simulink model "pendulo_optimo"  (R2017b)
settings: Solver=ode3  StartTime=0.0  StopTime=inf  FixedStep=h  RelTol=1e-3  EnableMultiTasking=on
values from neighbouring files (symbols this model uses):
  h = 0.001    [LQR_Ganancias.m]    (also in LQR_Ganancias2.m)
undefined symbols (not defined in the file or in its folder): National_Instruments, PCI
libraries: sldrtlib x4, fuzblock x1
settings Model: SimulationMode=external  Creator=Jovani  LastModifiedBy=js231
settings DataIOCC: LimitDataPoints=on  SaveFormat=Array
settings OptimizationCC: LifeSpan=inf
settings DebuggingCC: UnderspecifiedInitializationDetection=Classic  MergeDetectMultiDrivingBlocksExec=none  SolverPrmCheckMsg=warning  StateNameClashWarn=warning  SFUnexpectedBacktrackingDiag=warning  SFNoUnconditionalDefaultTransitionDiag=warning  SFExecutionAtInitializationDiag=none
settings HardwareCC: TargetBitPerLong=64  TargetBitPerPointer=64  TargetIntDivRoundTo=Zero  TargetEndianess=LittleEndian  TargetWordSize=64  TargetHWDeviceType=Intel->x86-64
settings ModelReferenceCC: PropagateSignalLabelsOutOfModel=off
settings RTWCC: SystemTargetFile=sldrt.tlc  TemplateMakefile=sldrt.tmf  Description=Simulink Desktop Real-Time  RTWCompilerOptimization=on
settings CodeAppCC: MaxIdLength=95  StateflowObjectComments=on
settings SimulinkDesktopRealTimeCC: TargetPreCompLibLocation=C:\Program Files\MATLAB\R2017b\toolbox\sldrt\lib\win64  TargetLangStandard=C89/C90 (ANSI)  SupportVariableSizeSignals=off
settings ConfigComp: CovMetricSettings=dw  CovHtmlReporting=on  CovSaveCumulativeToWorkspaceVar=on  CovSaveSingleToWorkspaceVar=on  CovExternalEMLEnable=off

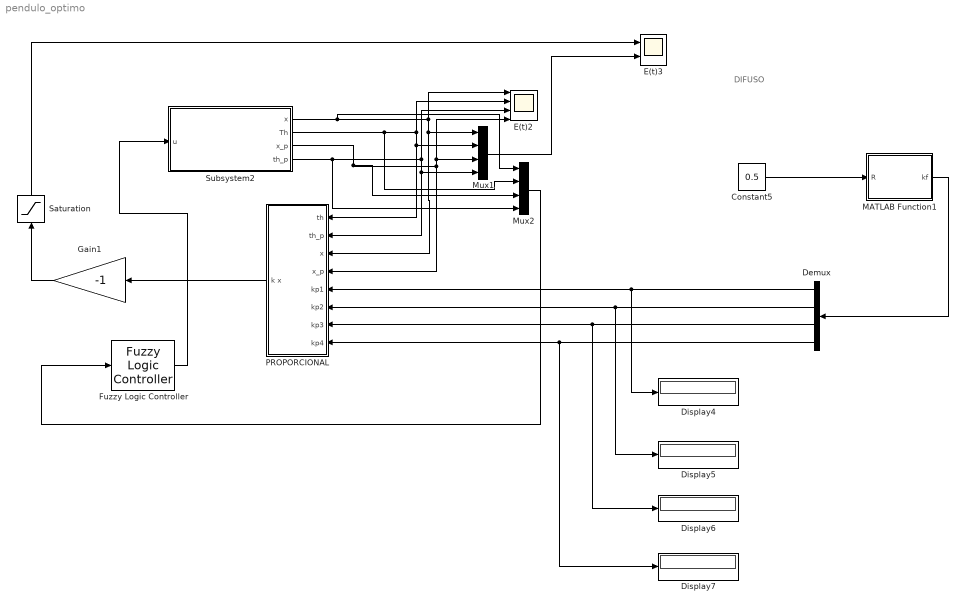
== system pendulo_optimo ==
  note: DIFUSO
  Constant5 : Constant  Value=0.5
  Demux : Demux
  Display{4..7} (4 alike) : Display
  E(t)2 : Scope  NumInputPorts=4
  E(t)3 : Scope  NumInputPorts=2
  Fuzzy Logic Controller : fuzblock/Fuzzy Logic  Controller  FIS=TS_carro_pendulo  OutputSampleNumber=101  DataType=double  FuzzifiedInputs=off  RuleFiringStrengths=off  RuleOutputs=off  AggregatedOutputs=off  SimulateUsing=Interpreted execution
  Gain1 : Gain  Gain=-1
  MATLAB Function1 : MATLAB Function  TreatAsAtomicUnit=on
  Mux1 : Mux
  Mux2 : Mux
  PROPORCIONAL : Subsystem
  Saturation : Saturate  UpperLimit=7.5  LowerLimit=-7.5
  Subsystem2 : Subsystem
  wires:
  Gain1/1 -> Saturation/1
  Subsystem2/4(th_p) -> Mux2/4, PROPORCIONAL/2(th_p), Mux1/4, E(t)2/3
  Subsystem2/3(x_p) -> Mux2/3, E(t)2/4, Mux1/3, PROPORCIONAL/4(x_p)
  Subsystem2/2(Th) -> Mux2/2, Mux1/2, PROPORCIONAL/1(th), E(t)2/2
  Subsystem2/1(x) -> Mux2/1, Mux1/1, PROPORCIONAL/3(x), E(t)2/1
  Mux1/1 -> E(t)3/2
  PROPORCIONAL/1(k x) -> Gain1/1
  Saturation/1 -> E(t)3/1
  Constant5/1 -> MATLAB Function1/1(R)
  MATLAB Function1/1(kf) -> Demux/1
  Demux/1 -> Display4/1, PROPORCIONAL/5(kp1)
  Demux/2 -> Display5/1, PROPORCIONAL/6(kp2)
  Demux/3 -> Display6/1, PROPORCIONAL/7(kp3)
  Demux/4 -> Display7/1, PROPORCIONAL/8(kp4)
  Mux2/1 -> Fuzzy Logic Controller/1
  Fuzzy Logic Controller/1 -> Subsystem2/1(u)

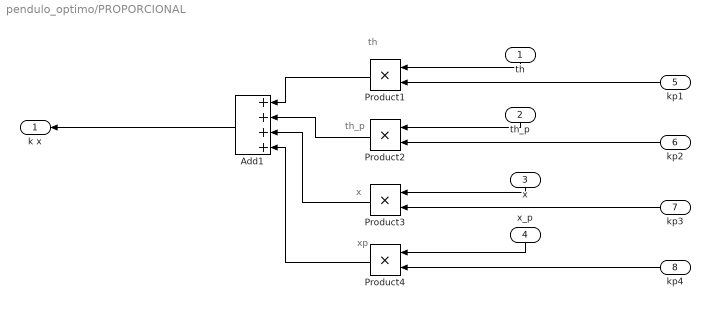
== system pendulo_optimo/PROPORCIONAL ==
  note: xp
  note: x
  note: th_p
  note: th
  th : Inport
  th_p : Inport  Port=2
  x : Inport  Port=3
  x_p : Inport  Port=4
  kp1 : Inport  Port=5
  kp2 : Inport  Port=6
  kp3 : Inport  Port=7
  kp4 : Inport  Port=8
  Add1 : Sum  Inputs=++++
  Product{1..4} (4 alike) : Product
  k x : Outport
  wires:
  x_p/1 -> Product4/1
  x/1 -> Product3/1
  th_p/1 -> Product2/1
  th/1 -> Product1/1
  Add1/1 -> k x/1
  Product4/1 -> Add1/4
  Product3/1 -> Add1/3
  Product2/1 -> Add1/2
  Product1/1 -> Add1/1
  kp3/1 -> Product3/2
  kp1/1 -> Product1/2
  kp2/1 -> Product2/2
  kp4/1 -> Product4/2

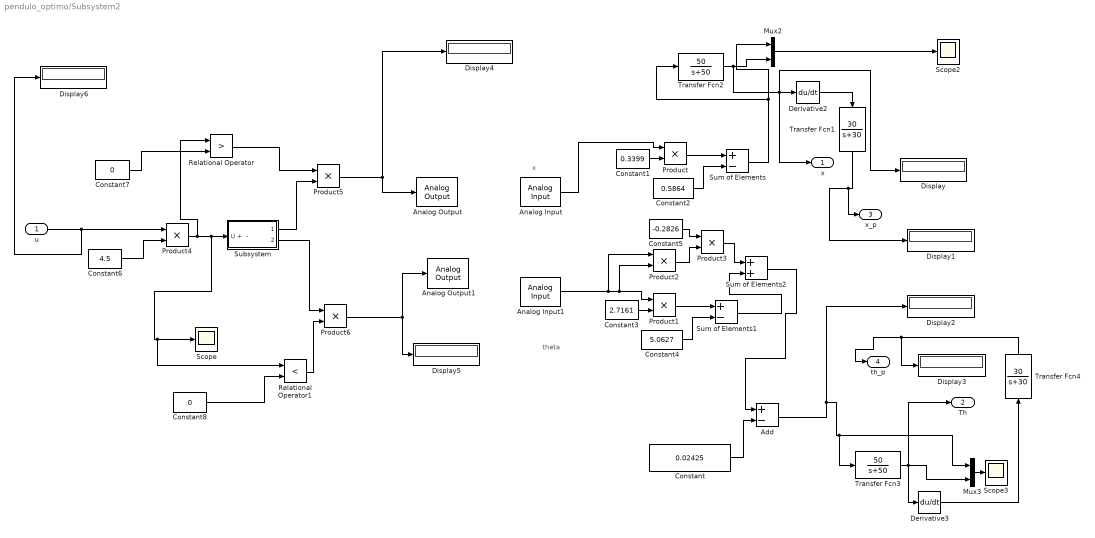
== system pendulo_optimo/Subsystem2 ==
  note: x
  note: theta
  u : Inport
  Add : Sum  Inputs=+-
  Analog Input : sldrtlib/Analog Input  SampleTime=h  MaxMissedTicks=10  ShowMissedTicks=off  YieldWhenWaiting=off  DrvName=National_Instruments/PCI-6071E  DrvAddress=0  DrvOptions=[0 0 0 0 0 0]  Channels=1  RangeMode=1  VoltRange=10  DataType=1
      settings: AttributesFormatString=National Instruments\nPCI-6071E [0h]  SourceProductName=Simulink Desktop Real-Time
  Analog Input1 : sldrtlib/Analog Input  SampleTime=h  MaxMissedTicks=10  ShowMissedTicks=off  YieldWhenWaiting=off  DrvName=National_Instruments/PCI-6071E  DrvAddress=0  DrvOptions=[0 0 0 0 0 0]  Channels=2  RangeMode=1  VoltRange=10  DataType=1
      settings: AttributesFormatString=National Instruments\nPCI-6071E [0h]  SourceProductName=Simulink Desktop Real-Time
  Analog Output : sldrtlib/Analog Output  SampleTime=h  MaxMissedTicks=10  ShowMissedTicks=off  YieldWhenWaiting=off  DrvName=National_Instruments/PCI-6071E  DrvAddress=0  DrvOptions=[0 0 0 0 0 0]  Channels=1  RangeMode=1  VoltRange=1  InitialValue=[]  FinalValue=[]
      settings: AttributesFormatString=National Instruments\nPCI-6071E [0h]  SourceProductName=Simulink Desktop Real-Time
  Analog Output1 : sldrtlib/Analog Output  SampleTime=h  MaxMissedTicks=10  ShowMissedTicks=off  YieldWhenWaiting=off  DrvName=National_Instruments/PCI-6071E  DrvAddress=0  DrvOptions=[0 0 0 0 0 0]  Channels=2  RangeMode=1  VoltRange=1  InitialValue=[]  FinalValue=[]
      settings: AttributesFormatString=National Instruments\nPCI-6071E [0h]  SourceProductName=Simulink Desktop Real-Time
  Constant : Constant  Value=0.02425
  Constant1 : Constant  Value=0.3399
  Constant2 : Constant  Value=0.5864
  Constant3 : Constant  Value=2.7161
  Constant4 : Constant  Value=5.0627
  Constant5 : Constant  Value=-0.2826
  Constant6 : Constant  Value=4.5
  Constant7 : Constant  Value=0
  Constant8 : Constant  Value=0
  Derivative2 : Derivative
  Derivative3 : Derivative
  Display{,1..6} (7 alike) : Display
  Mux2 : Mux  Inputs=2
  Mux3 : Mux  Inputs=2
  Product{,1..6} (7 alike) : Product
  Relational Operator : RelationalOperator  Operator=>  OutDataTypeStr=boolean  RndMeth=Nearest
  Relational Operator1 : RelationalOperator  Operator=<  OutDataTypeStr=boolean  RndMeth=Nearest
  Scope : Scope
  Scope2 : Scope
  Scope3 : Scope
  Subsystem : Subsystem
  Sum of Elements : Sum  Inputs=+-
  Sum of Elements1 : Sum  Inputs=+-
  Sum of Elements2 : Sum
  Transfer Fcn1 : TransferFcn  Numerator=[30]  Denominator=[1 30]
  Transfer Fcn2 : TransferFcn  Numerator=[50]  Denominator=[1 50]
  Transfer Fcn3 : TransferFcn  Numerator=[50]  Denominator=[1 50]
  Transfer Fcn4 : TransferFcn  Numerator=[30]  Denominator=[1 30]
  x : Outport
  Th : Outport  Port=2
  x_p : Outport  Port=3
  th_p : Outport  Port=4
  wires:
  Transfer Fcn4/1 -> th_p/1, Display3/1
  Transfer Fcn1/1 -> x_p/1, Display1/1
  Transfer Fcn3/1 -> Mux3/2, Derivative3/1, Th/1
  Mux3/1 -> Scope3/1
  Transfer Fcn2/1 -> Mux2/2, Derivative2/1, Display/1, x/1
  Mux2/1 -> Scope2/1
  Derivative3/1 -> Transfer Fcn4/1
  Derivative2/1 -> Transfer Fcn1/1
  Subsystem/2(neg ++) -> Product6/1
  Subsystem/1(pos ++) -> Product5/2
  Constant/1 -> Add/2
  Sum of Elements2/1 -> Add/1
  Relational Operator/1 -> Product5/1
  Product6/1 -> Analog Output1/1, Display5/1
  Relational Operator1/1 -> Product6/2
  Constant8/1 -> Relational Operator1/2
  Product5/1 -> Display4/1, Analog Output/1
  Constant7/1 -> Relational Operator/2
  Product4/1 -> Subsystem/1(U +  -), Scope/1, Relational Operator1/1, Relational Operator/1
  Constant6/1 -> Product4/2
  u/1 -> Product4/1, Display6/1
  Sum of Elements1/1 -> Sum of Elements2/2
  Product3/1 -> Sum of Elements2/1
  Product2/1 -> Product3/2
  Constant5/1 -> Product3/1
  Constant4/1 -> Sum of Elements1/2
  Constant3/1 -> Product1/2
  Product1/1 -> Sum of Elements1/1
  Sum of Elements/1 -> Transfer Fcn2/1, Mux2/1
  Constant2/1 -> Sum of Elements/2
  Constant1/1 -> Product/2
  Product/1 -> Sum of Elements/1
  Analog Input/1 -> Product/1
  Analog Input1/1 -> Product1/1, Product2/2, Product2/1
  Add/1 -> Mux3/1, Transfer Fcn3/1, Display2/1

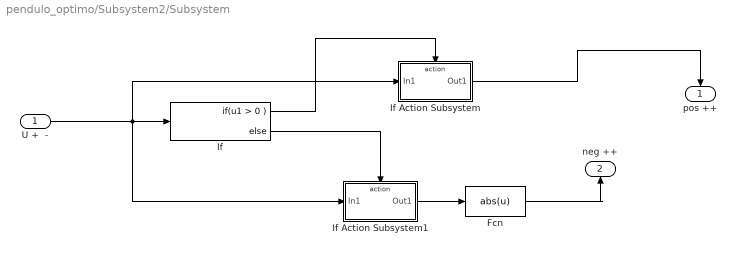
== system pendulo_optimo/Subsystem2/Subsystem ==
  U +  - : Inport
  Fcn : Fcn  Expr=abs(u)
  If : If  IfExpression=u1 > 0
  If Action Subsystem : Subsystem  TreatAsAtomicUnit=on
  If Action Subsystem1 : Subsystem  TreatAsAtomicUnit=on
  pos ++ : Outport
  neg ++ : Outport  Port=2
  wires:
  Fcn/1 -> neg ++/1
  If Action Subsystem1/1(Out1) -> Fcn/1
  If Action Subsystem/1(Out1) -> pos ++/1
  If/2 -> If Action Subsystem1/Action
  U +  -/1 -> If/1, If Action Subsystem/1(In1), If Action Subsystem1/1(In1)
  If/1 -> If Action Subsystem/Action

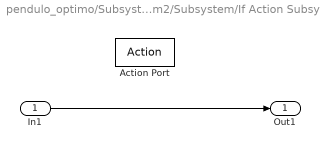
== system pendulo_optimo/Subsystem2/Subsystem/If Action Subsystem ==
  In1 : Inport
  Action Port : ActionPort  ActionType=then
  Out1 : Outport
  wires:
  In1/1 -> Out1/1

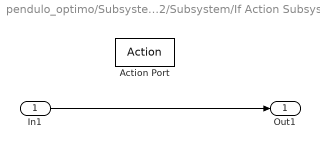
== system pendulo_optimo/Subsystem2/Subsystem/If Action Subsystem1 ==
  In1 : Inport
  Action Port : ActionPort  ActionType=else
  Out1 : Outport
  wires:
  In1/1 -> Out1/1

== matlab function pendulo_optimo/MATLAB Function1 ==
  data: R input; kf output
function kf = fcn(R)
%#codegen
%kf=[-60.1155,-15.6512,-6.3246,-10.4452];
kf=[-60.1155,-15.6512,-6.3246,-10.4452];

end
